simulink model "adc_zcu111"  (R2018a)
settings: Solver=VariableStepAuto  StartTime=0.0  StopTime=10.0  RelTol=1e-3
libraries: xbsIndex_r4 x2
settings Model: Creator=qwerty40  LastModifiedBy=qwerty40

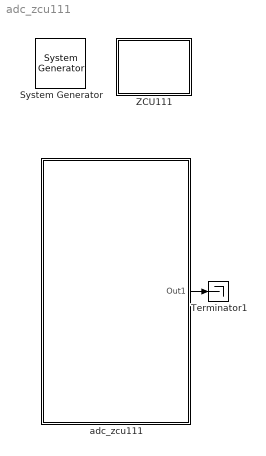
== system adc_zcu111 ==
  " System Generator" : xbsIndex_r4/ System Generator  Tag=genX  xilinxfamily=kintex7  part=xc7k325t  speed=-3  package=fbg676  synthesis_tool=Vivado  clock_wrapper=Clock Enables  directory=./netlist  proj_type=Vivado  Synth_file=Vivado Synthesis Defaults  Impl_file=Vivado Implementation Defaults  testbench=off  simulink_period=1  sysclk_period=10  dcm_input_clock_period=10  incr_netlist=off  trim_vbits=Everywhere in SubSystem  dbl_ovrd=According to Block Masks  core_generation=According to Block Masks  run_coregen=off  deprecated_control=off  eval_field=0  block_type=sysgen
  Terminator1 : Terminator
  ZCU111 : Subsystem  Tag=xps:xsg  mask(xsg core config){hw_sys=ZCU111:xczu28dr, clk_src=sys_clk, clk_rate=100, sample_period=1, synthesis_tool=XST}
      mask prompts: hw_sys "Hardware Platform"; clk_src "User IP Clock source"; clk_rate "User IP Clock Rate (MHz)"; sample_period "Sample Period"; synthesis_tool "Synthesis Tool:"
      mask help:
      | The XSG Core Config block is used to configure the System Generator design
      | for the casper_xps toolflow. Settings here are used to configure the
      | Xilinx System Generator block parameters automatically, and control toolflow
      | script  execution. It needs to be at the top level of all designs being compiled
      | with the casper_xps toolflow.
      mask init:
      | xps_xsg_zcu111_conf_mask;
      mask Help: eval('xlWeb([getenv(''MLIB_ROOT''), ''\doc\html\sys_xsg_core_config\sys_xsg_core_config.html''])')
      mask TypeOptions hw_sys: ZCU111:xczu28dr
      mask TypeOptions clk_src: sys_clk | adc_clk
      mask TypeOptions synthesis_tool: Leonardo Spectrum | Synplify | Synplify Pro | XST
      mask Display: fprintf(['ZCU111']);
  adc_zcu111 : Subsystem  Tag=xps:adc_zcu111  mask(adc_zcu111){tile_224_enable_pll=on, tile_224_sample_rate=4096, tile_224_clk_out=256.000, tile_224_ref_clk=512.000, tile_224_axi_stream_clk=0, adc_0=on, tile_224_adc0_digital_output=I/Q, tile_224_adc0_dec_mode=2x, tile_224_adc0_sample_per_cycle=8, tile_224_adc0_req_axis_clk=0, adc_1=on, tile_224_adc1_digital_output=I/Q, tile_224_adc1_dec_mode=2x, tile_224_adc1_sample_per_cycle=8, tile_224_adc1_req_axis_clk=0, tile_225_enable_pll=on, tile_225_sample_rate=4096, tile_225_clk_out=256.000, tile_225_ref_clk=512.000, tile_225_axi_stream_clk=0, adc_2=on, tile_225_adc0_digital_output=I/Q, tile_225_adc0_dec_mode=2x, tile_225_adc0_sample_per_cycle=8, tile_225_adc0_req_axis_clk=0, adc_3=on, tile_225_adc1_digital_output=I/Q, tile_225_adc1_dec_mode=2x, tile_225_adc1_sample_per_cycle=8, tile_225_adc1_req_axis_clk=0, tile_226_enable_pll=on, tile_226_sample_rate=4096, tile_226_clk_out=256.000, tile_226_ref_clk=512.000, tile_226_axi_stream_clk=0, adc_4=on, tile_226_adc0_digital_output=I/Q, tile_226_adc0_dec_mode=2x, tile_226_adc0_sample_per_cycle=8, tile_226_adc0_req_axis_clk=0, adc_5=on, tile_226_adc1_digital_output=I/Q, tile_226_adc1_dec_mode=2x, tile_226_adc1_sample_per_cycle=8, tile_226_adc1_req_axis_clk=0, tile_227_enable_pll=on, tile_227_sample_rate=4096, tile_227_clk_out=256.000, tile_227_ref_clk=512.000, tile_227_axi_stream_clk=0, adc_6=on, tile_227_adc0_digital_output=I/Q, tile_227_adc0_dec_mode=2x, tile_227_adc0_sample_per_cycle=8, tile_227_adc0_req_axis_clk=0, adc_7=on, tile_227_adc1_digital_output=I/Q, tile_227_adc1_dec_mode=2x, tile_227_adc1_sample_per_cycle=8, tile_227_adc1_req_axis_clk=0}
      mask prompts: tile_224_enable_pll "Enable PLL"; tile_224_sample_rate "Sampling Rate (MSPS)"; tile_224_clk_out "Clock Out (MHz)"; tile_224_ref_clk "Reference Clock (MHz)"; tile_224_axi_stream_clk "AXI4-Stream Clock (MHz)"; adc_0 "Enable ADC"; tile_224_adc0_digital_output "Digital Output Data"; tile_224_adc0_dec_mode "Decimation Mode"; tile_224_adc0_sample_per_cycle "Samples per AXI4-Stream Cycle"; adc_1 "Enable ADC"; tile_224_adc1_digital_output "Digital Output Data"; tile_224_adc1_dec_mode "Decimation Mode"; tile_224_adc1_sample_per_cycle "Samples per AXI4-Stream Cycle"; tile_225_enable_pll "Enable PLL"; tile_225_sample_rate "Sampling Rate (MSPS)"; tile_225_clk_out "Clock Out (MHz)"; tile_225_ref_clk "Reference Clock (MHz)"; tile_225_axi_stream_clk "AXI4-Stream Clock (MHz)"; adc_2 "Enable ADC"; tile_225_adc0_digital_output "Digital Output Data"; tile_225_adc0_dec_mode "Decimation Mode"; tile_225_adc0_sample_per_cycle "Samples per AXI4-Stream Cycle"; adc_3 "Enable ADC"; tile_225_adc1_digital_output "Digital Output Data"; tile_225_adc1_dec_mode "Decimation Mode"; tile_225_adc1_sample_per_cycle "Samples per AXI4-Stream Cycle"; tile_226_enable_pll "Enable PLL"; tile_226_sample_rate "Sampling Rate (MSPS)"; tile_226_clk_out "Clock Out (MHz)"; tile_226_ref_clk "Reference Clock (MHz)"; tile_226_axi_stream_clk "AXI4-Stream Clock (MHz)"; adc_4 "Enable ADC"; tile_226_adc0_digital_output "Digital Output Data"; tile_226_adc0_dec_mode "Decimation Mode"; tile_226_adc0_sample_per_cycle "Samples per AXI4-Stream Cycle"; adc_5 "Enable ADC"; tile_226_adc1_digital_output "Digital Output Data"; tile_226_adc1_dec_mode "Decimation Mode"; tile_226_adc1_sample_per_cycle "Samples per AXI4-Stream Cycle"; tile_227_enable_pll "Enable PLL"; tile_227_sample_rate "Sampling Rate (MSPS)"; tile_227_clk_out "Clock Out (MHz)"; tile_227_ref_clk "Reference Clock (MHz)"; tile_227_axi_stream_clk "AXI4-Stream Clock (MHz)"; adc_6 "Enable ADC"; tile_227_adc0_digital_output "Digital Output Data"; tile_227_adc0_dec_mode "Decimation Mode"; tile_227_adc0_sample_per_cycle "Samples per AXI4-Stream Cycle"; adc_7 "Enable ADC"; tile_227_adc1_digital_output "Digital Output Data"; tile_227_adc1_dec_mode "Decimation Mode"; tile_227_adc1_sample_per_cycle "Samples per AXI4-Stream Cycle"
      mask init:
      | %adc_zcu111_mask;
      mask Help: eval('xlWeb([getenv(''MLIB_ROOT''), ''\doc\html\adc_zcu111\adc_zcu111.html''])')
      mask TypeOptions tile_224_clk_out: 32.000 | 64.000 | 128.000 | 256.000
      mask TypeOptions tile_224_ref_clk: 103.261 | 104.136 | 105.026 | 105.931 | 106.852 | 107.790 | 108.743 | 109.714 | 110.703 | 111.709 | 112.734 | 113.778 | 114.841 | 115.925 | 117.029 | 118.154 | 119.301 | 120.471 | 121.663 | 122.880 | 124.121 | 125.388 | 126.680 | 128.000 | 129.347 | 130.723 | 132.129 | 133.565 | 135.033 | 136.533 | 138.067 | 139.636 | 141.241 | 142.884 | 144.565 | 146.286 | 148.048 | 149.854 | 151.704 | 153.600 | 155.544 | 157.539 | 159.584 | 161.684 | 163.840 | 166.054 | 168.329 | 170.667 | 173.070 | 175.543 | 178.087 | 180.706 | 183.403 | 186.182 | 189.046 | 192.000 | 195.048 | 198.194 | 201.443 | 204.800 | 208.271 | 211.862 | 215.579 | 219.429 | 223.418 | 227.556 | 231.849 | 236.308 | 240.941 | 245.760 | 250.776 | 256.000 | 261.447 | 267.130 | 273.067 | 279.273 | 285.767 | 292.571 | 299.707 | 307.200 | 315.077 | 323.368 | 332.108 | 341.333 | 351.086 | 361.412 | 372.364 | 384.000 | 396.387 | 409.600 | 423.724 | 438.857 | 455.111 | 472.615 | 491.520 | 512.000 | 534.261 | 558.546 | 585.143 | 614.400 | 646.737 | 682.667 | 722.824 | 768.000
      mask TypeOptions tile_224_adc0_digital_output: I/Q | Real
      mask TypeOptions tile_224_adc0_dec_mode: 1x | 2x | 4x | 8x
      mask TypeOptions tile_224_adc0_sample_per_cycle: 1 | 2 | 3 | 4 | 5 | 6 | 7 | 8
      mask TypeOptions tile_224_adc1_digital_output: I/Q | Real
      mask TypeOptions tile_224_adc1_dec_mode: 1x | 2x | 4x | 8x
      mask TypeOptions tile_224_adc1_sample_per_cycle: 1 | 2 | 3 | 4 | 5 | 6 | 7 | 8
      mask TypeOptions tile_225_clk_out: 32.000 | 64.000 | 128.000 | 256.000
      mask TypeOptions tile_225_ref_clk: 103.261 | 104.136 | 105.026 | 105.931 | 106.852 | 107.790 | 108.743 | 109.714 | 110.703 | 111.709 | 112.734 | 113.778 | 114.841 | 115.925 | 117.029 | 118.154 | 119.301 | 120.471 | 121.663 | 122.880 | 124.121 | 125.388 | 126.680 | 128.000 | 129.347 | 130.723 | 132.129 | 133.565 | 135.033 | 136.533 | 138.067 | 139.636 | 141.241 | 142.884 | 144.565 | 146.286 | 148.048 | 149.854 | 151.704 | 153.600 | 155.544 | 157.539 | 159.584 | 161.684 | 163.840 | 166.054 | 168.329 | 170.667 | 173.070 | 175.543 | 178.087 | 180.706 | 183.403 | 186.182 | 189.046 | 192.000 | 195.048 | 198.194 | 201.443 | 204.800 | 208.271 | 211.862 | 215.579 | 219.429 | 223.418 | 227.556 | 231.849 | 236.308 | 240.941 | 245.760 | 250.776 | 256.000 | 261.447 | 267.130 | 273.067 | 279.273 | 285.767 | 292.571 | 299.707 | 307.200 | 315.077 | 323.368 | 332.108 | 341.333 | 351.086 | 361.412 | 372.364 | 384.000 | 396.387 | 409.600 | 423.724 | 438.857 | 455.111 | 472.615 | 491.520 | 512.000 | 534.261 | 558.546 | 585.143 | 614.400 | 646.737 | 682.667 | 722.824 | 768.000
      mask TypeOptions tile_225_adc0_digital_output: I/Q | Real
      mask TypeOptions tile_225_adc0_dec_mode: 1x | 2x | 4x | 8x
      mask TypeOptions tile_225_adc0_sample_per_cycle: 1 | 2 | 3 | 4 | 5 | 6 | 7 | 8
      mask TypeOptions tile_225_adc1_digital_output: I/Q | Real
      mask TypeOptions tile_225_adc1_dec_mode: 1x | 2x | 4x | 8x
      mask TypeOptions tile_225_adc1_sample_per_cycle: 1 | 2 | 3 | 4 | 5 | 6 | 7 | 8
      mask TypeOptions tile_226_clk_out: 32.000 | 64.000 | 128.000 | 256.000
      mask TypeOptions tile_226_ref_clk: 103.261 | 104.136 | 105.026 | 105.931 | 106.852 | 107.790 | 108.743 | 109.714 | 110.703 | 111.709 | 112.734 | 113.778 | 114.841 | 115.925 | 117.029 | 118.154 | 119.301 | 120.471 | 121.663 | 122.880 | 124.121 | 125.388 | 126.680 | 128.000 | 129.347 | 130.723 | 132.129 | 133.565 | 135.033 | 136.533 | 138.067 | 139.636 | 141.241 | 142.884 | 144.565 | 146.286 | 148.048 | 149.854 | 151.704 | 153.600 | 155.544 | 157.539 | 159.584 | 161.684 | 163.840 | 166.054 | 168.329 | 170.667 | 173.070 | 175.543 | 178.087 | 180.706 | 183.403 | 186.182 | 189.046 | 192.000 | 195.048 | 198.194 | 201.443 | 204.800 | 208.271 | 211.862 | 215.579 | 219.429 | 223.418 | 227.556 | 231.849 | 236.308 | 240.941 | 245.760 | 250.776 | 256.000 | 261.447 | 267.130 | 273.067 | 279.273 | 285.767 | 292.571 | 299.707 | 307.200 | 315.077 | 323.368 | 332.108 | 341.333 | 351.086 | 361.412 | 372.364 | 384.000 | 396.387 | 409.600 | 423.724 | 438.857 | 455.111 | 472.615 | 491.520 | 512.000 | 534.261 | 558.546 | 585.143 | 614.400 | 646.737 | 682.667 | 722.824 | 768.000
      mask TypeOptions tile_226_adc0_digital_output: I/Q | Real
      mask TypeOptions tile_226_adc0_dec_mode: 1x | 2x | 4x | 8x
      mask TypeOptions tile_226_adc0_sample_per_cycle: 1 | 2 | 3 | 4 | 5 | 6 | 7 | 8
      mask TypeOptions tile_226_adc1_digital_output: I/Q | Real
      mask TypeOptions tile_226_adc1_dec_mode: 1x | 2x | 4x | 8x
      mask TypeOptions tile_226_adc1_sample_per_cycle: 1 | 2 | 3 | 4 | 5 | 6 | 7 | 8
      mask TypeOptions tile_227_clk_out: 32.000 | 64.000 | 128.000 | 256.000
      mask TypeOptions tile_227_ref_clk: 103.261 | 104.136 | 105.026 | 105.931 | 106.852 | 107.790 | 108.743 | 109.714 | 110.703 | 111.709 | 112.734 | 113.778 | 114.841 | 115.925 | 117.029 | 118.154 | 119.301 | 120.471 | 121.663 | 122.880 | 124.121 | 125.388 | 126.680 | 128.000 | 129.347 | 130.723 | 132.129 | 133.565 | 135.033 | 136.533 | 138.067 | 139.636 | 141.241 | 142.884 | 144.565 | 146.286 | 148.048 | 149.854 | 151.704 | 153.600 | 155.544 | 157.539 | 159.584 | 161.684 | 163.840 | 166.054 | 168.329 | 170.667 | 173.070 | 175.543 | 178.087 | 180.706 | 183.403 | 186.182 | 189.046 | 192.000 | 195.048 | 198.194 | 201.443 | 204.800 | 208.271 | 211.862 | 215.579 | 219.429 | 223.418 | 227.556 | 231.849 | 236.308 | 240.941 | 245.760 | 250.776 | 256.000 | 261.447 | 267.130 | 273.067 | 279.273 | 285.767 | 292.571 | 299.707 | 307.200 | 315.077 | 323.368 | 332.108 | 341.333 | 351.086 | 361.412 | 372.364 | 384.000 | 396.387 | 409.600 | 423.724 | 438.857 | 455.111 | 472.615 | 491.520 | 512.000 | 534.261 | 558.546 | 585.143 | 614.400 | 646.737 | 682.667 | 722.824 | 768.000
      mask TypeOptions tile_227_adc0_digital_output: I/Q | Real
      mask TypeOptions tile_227_adc0_dec_mode: 1x | 2x | 4x | 8x
      mask TypeOptions tile_227_adc0_sample_per_cycle: 1 | 2 | 3 | 4 | 5 | 6 | 7 | 8
      mask TypeOptions tile_227_adc1_digital_output: I/Q | Real
      mask TypeOptions tile_227_adc1_dec_mode: 1x | 2x | 4x | 8x
      mask TypeOptions tile_227_adc1_sample_per_cycle: 1 | 2 | 3 | 4 | 5 | 6 | 7 | 8
      mask DialogControl adc_tile_224 Prompt: ADC Tile 224
      mask DialogControl pll_clocking_config_224 Prompt: PLL and Clocking Configuration
      mask DialogControl tile_224_adc0 Prompt: ADC 0
      mask DialogControl tile_224_adc0_data_settings Prompt: Data Settings
      mask DialogControl tile_224_adc0_req_axis_clk_label Prompt: Required AXI4-Stream clock:
      mask DialogControl tile_224_adc1 Prompt: ADC 1
      mask DialogControl tile_224_adc1_data_settings Prompt: Data Settings
      mask DialogControl tile_224_adc1_req_axis_clk_label Prompt: Required AXI4-Stream clock:
      mask DialogControl adc_tile_225 Prompt: ADC Tile 225
      mask DialogControl pll_clocking_config_225 Prompt: PLL and Clocking Configuration
      mask DialogControl tile_225_adc0 Prompt: ADC 0
      mask DialogControl tile_225_adc0_data_settings Prompt: Data Settings
      mask DialogControl tile_225_adc0_req_axis_clk_label Prompt: Required AXI4-Stream clock:
      mask DialogControl tile_225_adc1 Prompt: ADC 1
      mask DialogControl tile_225_adc1_data_settings Prompt: Data Settings
      mask DialogControl tile_225_adc1_req_axis_clk_label Prompt: Required AXI4-Stream clock:
      mask DialogControl adc_tile_226 Prompt: ADC Tile 226
      mask DialogControl pll_clocking_config_226 Prompt: PLL and Clocking Configuration
      mask DialogControl tile_226_adc0 Prompt: ADC 0
      mask DialogControl tile_226_adc0_data_settings Prompt: Data Settings
      mask DialogControl tile_226_adc0_req_axis_clk_label Prompt: Required AXI4-Stream clock:
      mask DialogControl tile_226_adc1 Prompt: ADC 1
      mask DialogControl tile_226_adc1_data_settings Prompt: Data Settings
      mask DialogControl tile_226_adc1_req_axis_clk_label Prompt: Required AXI4-Stream clock:
      mask DialogControl adc_tile_227 Prompt: ADC Tile 227
      mask DialogControl pll_clocking_config_227 Prompt: PLL and Clocking Configuration
      mask DialogControl tile_227_adc0 Prompt: ADC 0
      mask DialogControl tile_227_adc0_data_settings Prompt: Data Settings
      mask DialogControl tile_227_adc0_req_axis_clk_label Prompt: Required AXI4-Stream clock:
      mask DialogControl tile_227_adc1 Prompt: ADC 1
      mask DialogControl tile_227_adc1_data_settings Prompt: Data Settings
      mask DialogControl tile_227_adc1_req_axis_clk_label Prompt: Required AXI4-Stream clock:
  wires:
  adc_zcu111/1(Out1) -> Terminator1/1

== system adc_zcu111/ZCU111 ==

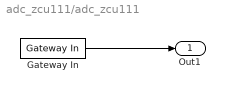
== system adc_zcu111/adc_zcu111 ==
  Gateway In : xbsIndex_r4/Gateway In  gui_display_data_type=Fixed-point  arith_type="Signed  (2's comp)"  n_bits=16  bin_pt=14  preci_type=Single  exp_width=8  frac_width=24  rows=1  columns=1  quantization="Round  (unbiased: +/- Inf)"  overflow=Saturate  period=1  UseAsADC=off  ADCChannel='1'  interface=None  automatic_assignment=on  address_offset=hex2dec('00')  intf_name=''  intf_description=''  default_value=0  timing_constraint=None  locs_specified=off  LOCs={}  io_standard={}  inherit_from_input=off  hdl_port=on  dbl_ovrd=off  block_type=gatewayin
  Out1 : Outport
  wires:
  Gateway In/1 -> Out1/1
